simulink model "sgMdl_IO133_Loopback"  (R2024b)
settings: Solver=FixedStepAuto  StartTime=0.0  StopTime=inf  RelTol=1e-3  EnableMultiTasking=on
libraries: speedgoatlib_IO133 x5
Description:
  | IO133 - Analog and Digital Loopback
settings Model: sg_rtwmakecfg_data=_sglibc_  ModifiedByFormat=Speedgoat  SimulationMode=external  ExtModeTrigDuration=100000  Creator=Speedgoat  LastModifiedBy=Speedgoat
settings SolverCC: ConcurrentTasks=on  AlgebraicLoopSolver=TrustRegion  PositivePriorityOrder=on  AutoInsertRateTranBlk=on  InsertRTBMode=Never (minimum delay)
settings DataIOCC: SaveFormat=StructureWithTime  ReturnWorkspaceOutputs=off
settings OptimizationCC: BlockReduction=off  OptimizeBlockIOStorage=off  BufferReuse=off  GlobalBufferReuse=off  ExpressionFolding=off  LocalBlockOutputs=off
settings DebuggingCC: TasksWithSamePriorityMsg=none  UnconnectedInputMsg=warning  UnconnectedOutputMsg=warning  UnconnectedLineMsg=warning  SFExecutionAtInitializationDiag=none  ArithmeticOperatorsInVariantConditions=warning
settings HardwareCC: ProdBitPerLong=64  ProdLongLongMode=on  ProdHWDeviceType=Intel->x86-64 (Linux 64)
settings ModelReferenceCC: EnableRefExpFcnMdlSchedulingChecks=on
settings SFSimCC: SimUseLocalCustomCode=off  CustomCodeUndefinedFunction=UseInterfaceOnly
settings RTWCC: Description=Speedgoat Real-Time Target Machine  SystemTargetFile=speedgoat.tlc  TemplateMakefile=slrealtime_default_tmf  RTWUseLocalCustomCode=off  Toolchain=Simulink Real-Time Toolchain  BuildConfiguration=Faster Runs  TargetLang=C++  GPUComputeCapability=3.5  DLArmComputeVersion=19.05
settings CodeAppCC: StateflowObjectComments=on
settings SimulinkRealTimeTargetCC: SubcomponentCodeInterfacePackaging=Reusable function  InstructionSetFMA=off  LogToMDFFile=off  SLRTFileLogMaxRuns=10  UseGCCFastMath=on
settings ConfigComp: CovBoundaryAbsTol=1.0e-5

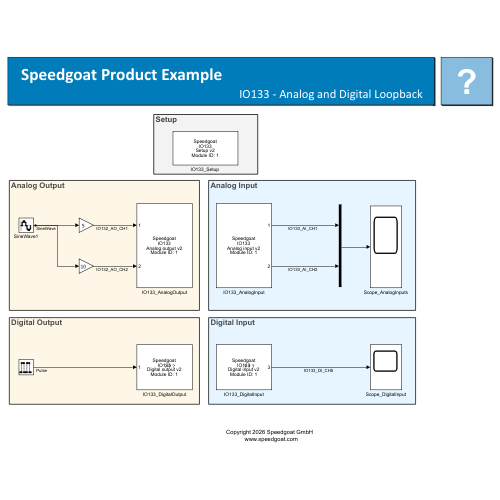
[thumbnail: Simulink's stored preview of the top-level diagram]
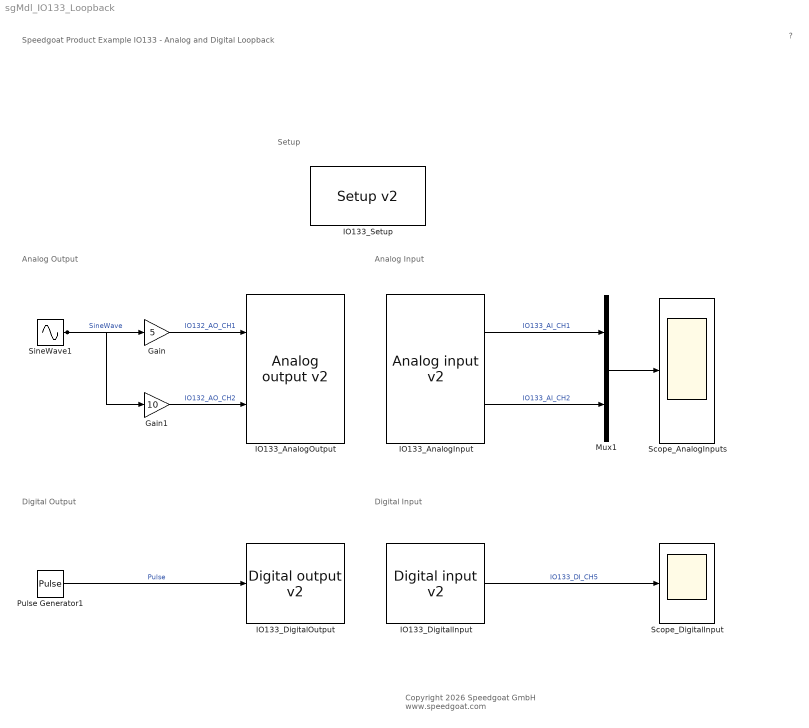
== system sgMdl_IO133_Loopback ==
  note: Setup
  note: Analog Input
  note: Digital Output
  note: Analog Output
  note: Digital Input
  note: Speedgoat Product Example
      | IO133 - Analog and Digital Loopback
  note: ?
  note: Copyright 2026 Speedgoat GmbH
      |  www.speedgoat.com
  Gain : Gain  Gain=5
  Gain1 : Gain  Gain=10
  IO133_AnalogInput : speedgoatlib_IO133/Analog input v2   parModuleId=1  parSampleTime=0.001  parPciSlot=-1  parAdcChannels=[1 2]  parAdcVoltageRange=[2 2]  parAdcOversamplRate=[1 1]  parAdcContSampling=0  parAdcDmaEnable=0  parAdcActiveDmaDevices=[1 1]  parAdcFrameSize=100
      settings: SourceProductName=Simulink Real-Time: Speedgoat I/O Driver Library
  IO133_AnalogOutput : speedgoatlib_IO133/Analog output v2   parModuleId=1  parSampleTime=0.001  parPciSlot=-1  parDacChannels=[1 2]  parDacVoltageRange=[5 5 6 6 5 5 5 5]  parDacInitValues=[0 0]  parDacReset=[1 1]  parDacSyncOut=1  parDacDmaEnable=0  parDacActiveDmaDevices=[1 1]  parDacDmaLatency=2  parDacFrameSize=100
      settings: SourceProductName=Simulink Real-Time: Speedgoat I/O Driver Library
  IO133_DigitalInput : speedgoatlib_IO133/Digital input v2   parModuleId=1  parSampleTime=0.001  parPciSlot=-1  parDiChannels=5
      settings: SourceProductName=Simulink Real-Time: Speedgoat I/O Driver Library
  IO133_DigitalOutput : speedgoatlib_IO133/Digital output v2   parModuleId=1  parSampleTime=0.001  parPciSlot=-1  parDoChannels=1  parDoInitValues=0  parDoReset=1
      settings: SourceProductName=Simulink Real-Time: Speedgoat I/O Driver Library
  "IO133_Setup " : speedgoatlib_IO133/Setup v2   parPciSlot=-1  parModuleId=1  parInterModuleSync=None  parConvClockBaseRate=20MHz  parConvClock1Divider=20000  parConvClock2Divider=20000  parFrameTriggerEnable=off  parFrameTriggerDivider=10  parConvClock1BaseRate=1  parConvClock2BaseRate=1  parFrameTriggerClock=1  parAdcChannels=[1 2]  parAdcRange1=+-10V  parAdcRange2=+-10V  parAdcVoltageRange=[2 2]  parAdcOversampling1=None  parAdcOversampling2=None  parAdcOversamplRate=[1 1]  parAdcContSampling=off  parAdcDataCorrection=Automatic  parAdcCorrectionActive={}  parAdcCorrectionPm5V={'1','0','0';'2','0','0';'3','0','0';'4','0','0';'5','0','0';'6','0','0';'7','0','0';'8','0','0';'9','0','0';'10','0','0';'11','0','0';'12','0','0';'13','0','0';'14','0','0';'15','0','0';'16','0','0'}  parAdcCorrectionPm10V={'1','0','0';'2','0','0';'3','0','0';'4','0','0';'5','0','0';'6','0','0';'7','0','0';'8','0','0';'9','0','0';'10','0','0';'11','0','0';'12','0','0';'13','0','0';'14','0','0';'15','0','0';'16','0','0'}  parAdcDmaEnable=off  parAdcDmaClock=Clock 1  parAdcFrameSize_=100  parAdcSampleTime_=-1  parAdcActiveDmaDevices=[1 1]  parAdcFrameTriggerEnable=0  parAdcFrameSize=100  parAdcSampleTime=0.1  parDacChannels=[1 2]  parDacInitValues=0  parDacReset=1  parDacRange1=+-10V  parDacRange2=+-10V  parDacRange3=+-10.8V  parDacRange4=+-10.8V  parDacRange5=+-10V  parDacRange6=+-10V  parDacRange7=+-10V  parDacRange8=+-10V  parDacVoltageRange=[5 5 6 6 5 5 5 5]  parDacSyncOut=on  parDacDataCorrection=Automatic  parDacCorrectionActive={}  parDacCorrection5V={'1','0','0';'2','0','0';'3','0','0';'4','0','0';'5','0','0';'6','0','0';'7','0','0';'8','0','0'}  parDacCorrection10V={'1','0','0';'2','0','0';'3','0','0';'4','0','0';'5','0','0';'6','0','0';'7','0','0';'8','0','0'}  parDacCorrection10_8V={'1','0','0';'2','0','0';'3','0','0';'4','0','0';'5','0','0';'6','0','0';'7','0','0';'8','0','0'}  parDacCorrectionPm5V={'1','0','0';'2','0','0';'3','0','0';'4','0','0';'5','0','0';'6','0','0';'7','0','0';'8','0','0'}  parDacCorrectionPm10V={'1','0','0';'2','0','0';'3','0','0';'4','0','0';'5','0','0';'6','0','0';'7','0','0';'8','0','0'}  parDacCorrectionPm10_8V={'1','0','0';'2','0','0';'3','0','0';'4','0','0';'5','0','0';'6','0','0';'7','0','0';'8','0','0'}  parDacDmaEnable=off  parDacDmaLatency=Until next frame  parDacDmaClock=Clock 1  parDacFrameSize_=100  parDacSampleTime_=-1  parDacActiveDmaDevices=[1 1]  parDacFrameTriggerEnable=0  parDacFrameSize=100  parDacSampleTime=0.1  parDoChannels=[1]  parDoInitValues=0  parDoReset=1  parDiChannels=[5]  parDiDebounceEnable=off  parDiDebounceTime=0  parDiDebounceValue=0  parDioPullRefFront=Pull-up 3.3V  parDioPullRefRear=Floating
      settings: SourceProductName=Simulink Real-Time: Speedgoat I/O Driver Library
  Mux1 : Mux  Inputs=2
  Pulse Generator1 : DiscretePulseGenerator  Period=10  PulseWidth=5  SampleTime=0.001
  Scope_AnalogInputs : Scope
  Scope_DigitalInput : Scope
  SineWave1 : Sin  Frequency=2*pi  Samples=50  SampleTime=0.001
  wires:
  SineWave1/1 -> Gain/1, Gain1/1  "SineWave"
  Gain/1 -> IO133_AnalogOutput/1  "IO132_AO_CH1"
  Gain1/1 -> IO133_AnalogOutput/2  "IO132_AO_CH2"
  Mux1/1 -> Scope_AnalogInputs/1
  IO133_AnalogInput/2 -> Mux1/2  "IO133_AI_CH2"
  IO133_AnalogInput/1 -> Mux1/1  "IO133_AI_CH1"
  Pulse Generator1/1 -> IO133_DigitalOutput/1  "Pulse"
  IO133_DigitalInput/1 -> Scope_DigitalInput/1  "IO133_DI_CH5"
